simulink model "playback_data"  (R2015a)
settings: Solver=FixedStepDiscrete  SolverMode=SingleTasking  StartTime=76  StopTime=110  FixedStep=sample_time  RelTol=1e-3
undefined symbols (not defined in the file): A1_notch_f1, A2_notch_f1, A_kalman_swing_load, A_kalman_transverse, A_kalman_vertical, A_lpf_accelerometer, A_lpf_dtau, A_lpf_fourbar_angles, A_lpf_imu, A_lpf_lateral_angle, B1_lpf_accelerometer, B1_lpf_dtau, B1_lpf_fourbar_angles, B1_lpf_imu, B1_lpf_lateral_angle, B1_notch_f1, B2_lpf_accelerometer, B2_lpf_dtau, B2_lpf_fourbar_angles, B2_lpf_imu, B2_lpf_lateral_angle, B2_notch_f1, B_dx_versus_x0, B_kalman_swing_load, B_kalman_transverse, B_kalman_vertical, backwards_K_sag_of_t, backwards_P_sag_of_t, C_kalman_swing_load, C_kalman_transverse, C_kalman_vertical, com_leg_motor, com_torso, contact_threshold, control_start_time, d_ankle_to_foot, d_vertical_com, desired_com_forward_velocity, desired_com_lateral_velocity, desired_initial_leg_roll_left, desired_initial_leg_roll_right, desired_stance_beta2, desired_standing_torso_pitch, desired_standing_torso_roll, desired_standing_z, desired_torso_pitch, desired_torso_roll, Discrete, enable_bouncing, fcut_contact, fdesignblkfcn, forward_dx_of_dxstar, forward_x_of_dxstar, g, gcbh, HIP_MTR_MAX_CONT_TORQUE, HIP_MTR_MAX_TORQUE, i_leg_motor, i_robot, i_torso ... (+78)
libraries: simulink x65, dsparch4 x18, ctrlSharedLib x14, dspfdesign x4
(part 11 of 13)

== matlab function playback_data/Control1/Behavior Control/Primary and Lateral Behavior/Desired Forward Velocity ==
  data: dx_takeoff input; desired_dx output; desired_forward_velocity input; forward_velocity_target_step parameter
function desired_dx = dx_command(dx_takeoff, desired_forward_velocity, forward_velocity_target_step)
    desired_direction = sign(desired_forward_velocity);
    desired_dx = dx_takeoff + desired_direction*forward_velocity_target_step;
    desired_dx = max(min(desired_dx, abs(desired_forward_velocity)),-abs(desired_forward_velocity));
end

== matlab function playback_data/Control1/Behavior Control/Primary and Lateral Behavior/Flight/Avoid Hitting Mechanical Limits ==
  data: back_cmd output double; front_cmd output double; dback_cmd output double; dfront_cmd output double; ddback_cmd output double; ddfront_cmd output double; back_desired input; dback_desired input; ddback_desired input; front_desired input; dfront_desired input; ddfront_desired input; min_front_bar_angle parameter; max_front_bar_angle parameter; min_back_bar_angle parameter; max_back_bar_angle parameter
%% Avoid joint limits by ensuring we don't command velocities/accelerations that would push us into them when we are close to them.
function [back_cmd, front_cmd, dback_cmd, dfront_cmd, ddback_cmd, ddfront_cmd] ...
    = AvoidFourbarLimits(back_desired,dback_desired, ddback_desired, ...
          front_desired, dfront_desired, ddfront_desired, ...
          min_front_bar_angle, max_front_bar_angle, min_back_bar_angle, max_back_bar_angle)
    [back_cmd, front_cmd, dback_cmd, dfront_cmd, ddback_cmd, ddfront_cmd] = AvoidFourbarLimits(back_desired,dback_desired, ddback_desired, front_desired, dfront_desired, ddfront_desired, min_front_bar_angle, max_front_bar_angle, min_back_bar_angle, max_back_bar_angle);
end

== matlab function playback_data/Control1/Behavior Control/Primary and Lateral Behavior/Flight/Avoid Virtual Leg Length Limits ==
  data: l_leg_desired input; dl_leg_desired input; ddl_leg_desired input; l_leg_cmd output double; dl_leg_cmd output double; ddl_leg_cmd output double; min_leg_length parameter; max_leg_length parameter
%% Avoid virtual leg length limits by ensuring we don't command position/velocities/accelerations that would hit them.
function [l_leg_cmd, dl_leg_cmd, ddl_leg_cmd] = AvoidVirtualLengthLimits(l_leg_desired, dl_leg_desired, ddl_leg_desired, min_leg_length, max_leg_length)
    [l_leg_cmd, dl_leg_cmd, ddl_leg_cmd] = AvoidVirtualLengthLimits(l_leg_desired, dl_leg_desired, ddl_leg_desired, min_leg_length, max_leg_length);
end

== matlab function playback_data/Control1/Behavior Control/Primary and Lateral Behavior/Flight/Calculate Time Until Touchdown ==
  data: z_dz input; t output; z_land parameter; g parameter
function t = EstimateTouchdown(z_dz, z_land, g)
  z_hat = z_dz(1); 
  dz_hat = z_dz(2);
  t = (-dz_hat-sqrt( max(dz_hat^2 - 4*g/2*(z_land-z_hat),0) ))/(-g);
end

== matlab function playback_data/Control/Behavior Control/Primary and Lateral Behavior/Closed Loop Compensation/ESTIMATE CLOSED LOOP ERROR Y FOR VARIABLE SPEED ==
  data: dx_land_hist input; A_cl output; delta_ux_hist input; dx_lift_hist input; dx_star_hist input; B_dx_versus_x0 parameter; W_real input; epsilon_0 output; c output; A_cl_nb output; epsilon_0_nb output; c_nb output
function [A_cl, epsilon_0, c, ...
          A_cl_nb, epsilon_0_nb, c_nb] = error_fitting_dxstar...
         (dx_land_hist, delta_ux_hist, dx_lift_hist, dx_star_hist,...
          B_dx_versus_x0, W_real)
% data_length = min([length(dx_lift_hist), filter_length]);
data_length = length(dx_lift_hist);
assert(data_length < 100);
% add fake data
fake_dx_land_err_magnitude = 0.1; fake_dx_star_magnitude = 0.1;
[fgrid_dx_land_err, fgrid_dx_star, fgrid_dx_lift_err] = ...
    meshgrid(fake_dx_land_err_magnitude*[-1 1],fake_dx_star_magnitude*[-1 1],0);
fake_data_length = numel(fgrid_dx_land_err);
fake_dx_land_err = fgrid_dx_land_err(:);
fake_dx_star = fgrid_dx_star(:);
fake_dx_lift_err = fgrid_dx_lift_err(:);
fake_delta_ux = zeros(fake_data_length,1);
% assert(fake_data_length<100);
% assert(filter_length<100);
% fake_dx_land_err = linspace(-0.1, 0.1, fake_data_length)';
% fake_dx_lift_err = zeros(fake_data_length,1);
% fake_delta_ux = zeros(fake_data_length,1);
% fake_dx_star = linspace(-0.25, 0.25, fake_data_length)';
dx_land_err = [reshape(dx_land_hist(1:data_length)-dx_star_hist(1:data_length),...
                       data_length, 1); fake_dx_land_err];
dx_lift_err = [reshape(dx_lift_hist(1:data_length)-dx_star_hist(1:data_length),...
                       data_length, 1); fake_dx_lift_err];
dx_star = [reshape(dx_star_hist(1:data_length), data_length,1); fake_dx_star];
delta_ux = [reshape(delta_ux_hist(1:data_length), data_length, 1); fake_delta_ux];
% weighted least squares
W = diag([W_real*ones(1,data_length), ones(1,fake_data_length)]);
Y = dx_lift_err - B_dx_versus_x0*delta_ux;
X = [dx_land_err, dx_star, ones(data_length+fake_data_length,1)];
% linear regression for s_{i+1}-s0 = A_cl*(s_i-s0) + epsilon_0 + c(s0) + B*delta_u
% solve for Y = X*beta, beta column vector
beta_hat = (X'*W*X)\X'*W*Y;
W_nobias = diag([W_real*ones(1,data_length), 0.001*ones(1,fake_data_length)]);
beta_hat_nobias = (X'*W_nobias*X)\X'*W_nobias*Y;
A_cl = beta_hat(1);
c = beta_hat(2);
epsilon_0 = beta_hat(3);
A_cl_nb = beta_hat_nobias(1);
c_nb = beta_hat_nobias(2);
epsilon_0_nb = beta_hat_nobias(3);

== matlab function playback_data/Control/Behavior Control/Primary and Lateral Behavior/Desired Forward Velocity ==
  data: dx_takeoff input; desired_dx output; desired_forward_velocity input; forward_velocity_target_step parameter
function desired_dx = dx_command(dx_takeoff, desired_forward_velocity, forward_velocity_target_step)
    desired_direction = sign(desired_forward_velocity);
    desired_dx = dx_takeoff + desired_direction*forward_velocity_target_step;
    desired_dx = max(min(desired_dx, abs(desired_forward_velocity)),-abs(desired_forward_velocity));
end

== matlab function playback_data/Control/Behavior Control/Primary and Lateral Behavior/Flight/Avoid Hitting Mechanical Limits ==
  data: back_cmd output double; front_cmd output double; dback_cmd output double; dfront_cmd output double; ddback_cmd output double; ddfront_cmd output double; back_desired input; dback_desired input; ddback_desired input; front_desired input; dfront_desired input; ddfront_desired input; min_front_bar_angle parameter; max_front_bar_angle parameter; min_back_bar_angle parameter; max_back_bar_angle parameter
%% Avoid joint limits by ensuring we don't command velocities/accelerations that would push us into them when we are close to them.
function [back_cmd, front_cmd, dback_cmd, dfront_cmd, ddback_cmd, ddfront_cmd] ...
    = AvoidFourbarLimits(back_desired,dback_desired, ddback_desired, ...
          front_desired, dfront_desired, ddfront_desired, ...
          min_front_bar_angle, max_front_bar_angle, min_back_bar_angle, max_back_bar_angle)
    [back_cmd, front_cmd, dback_cmd, dfront_cmd, ddback_cmd, ddfront_cmd] = AvoidFourbarLimits(back_desired,dback_desired, ddback_desired, front_desired, dfront_desired, ddfront_desired, min_front_bar_angle, max_front_bar_angle, min_back_bar_angle, max_back_bar_angle);
end

== matlab function playback_data/Control/Behavior Control/Primary and Lateral Behavior/Flight/Avoid Virtual Leg Length Limits ==
  data: l_leg_desired input; dl_leg_desired input; ddl_leg_desired input; l_leg_cmd output double; dl_leg_cmd output double; ddl_leg_cmd output double; min_leg_length parameter; max_leg_length parameter
%% Avoid virtual leg length limits by ensuring we don't command position/velocities/accelerations that would hit them.
function [l_leg_cmd, dl_leg_cmd, ddl_leg_cmd] = AvoidVirtualLengthLimits(l_leg_desired, dl_leg_desired, ddl_leg_desired, min_leg_length, max_leg_length)
    [l_leg_cmd, dl_leg_cmd, ddl_leg_cmd] = AvoidVirtualLengthLimits(l_leg_desired, dl_leg_desired, ddl_leg_desired, min_leg_length, max_leg_length);
end

== matlab function playback_data/Control/Behavior Control/Primary and Lateral Behavior/Flight/Calculate Time Until Touchdown ==
  data: z_dz input; t output; z_land parameter; g parameter
function t = EstimateTouchdown(z_dz, z_land, g)
  z_hat = z_dz(1); 
  dz_hat = z_dz(2);
  t = (-dz_hat-sqrt( max(dz_hat^2 - 4*g/2*(z_land-z_hat),0) ))/(-g);
end

== matlab function playback_data/Control1/Behavior Control/Primary and Lateral Behavior/Flight/Convert COM Position to Joint Angles + Leg Length  ==
  data: hopping input; desired_leg_length output; X_star input; Y_star input; Z_star input; right_left input; com_pelvis_body input; desired_alpha output; desired_beta output; dcom_pelvis_body input; roll input; pitch input; sagittal_angle input; lateral_angle input; leg_length input; lateral_offset parameter; desired_initial_leg_roll_right parameter; desired_initial_leg_roll_left parameter; d_vertical_com parameter; desired_standing_z parameter
function [ desired_leg_length, desired_alpha, desired_beta ]  =  ...
          ConvertToJointAnglesAndLegLength(hopping, X_star, Y_star, Z_star, right_left,...
                           com_pelvis_body, dcom_pelvis_body, ...
                           roll, pitch, sagittal_angle, lateral_angle, leg_length,...
                           lateral_offset, desired_initial_leg_roll_right, desired_initial_leg_roll_left, d_vertical_com, desired_standing_z) 

    q = [roll(1), pitch(1), sagittal_angle(1), lateral_angle(1), leg_length(1)];
    dq = [roll(2), pitch(2), sagittal_angle(2), lateral_angle(2), leg_length(2)];
    [desired_alpha, desired_beta, desired_leg_length]  =  ConvertComPositionToLegAnglesAndLegLength(X_star, Y_star, Z_star, right_left, com_pelvis_body, dcom_pelvis_body, q, dq, lateral_offset);   
                       
    if ~hopping
        desired_leg_length = [desired_standing_z-d_vertical_com; 0; 0];
        desired_alpha = [pi - pitch(1); -pitch(2); 0];
        desired_beta = [desired_initial_leg_roll_left; 0; 0];
        if right_left
            desired_beta = [desired_initial_leg_roll_right; 0; 0];
        end
    end
    
end

== matlab function playback_data/Control1/Behavior Control/Primary and Lateral Behavior/Flight/Generate Parabolic Foot Trajectories ==
  data: time_remaining input; est_duration input; x_star input; y_star input; x0 input; dx0 input; y0 input; dy0 input; zdz0 input; max_retract input; flight input; z_land parameter; min_f_duration parameter; X_star output size=3; Y_star output size=3; Z_star output size=3
%% Parabolic trajectory generation for x, y, and z
% est_duration: estimated flight time
% time_remaining: time until estimated touchdown
% stance: 1 if in stance, 0 otherwise
% x_star: desired x for foot to COM
% y_star: desired y for foot to COM
% x0: x position at takeoff
% y0: y position at takeoff
% zdz0: [z, dz] at takeoff
% max_retract: how high to lift z for ground clearance
% z_land: nominal z height for landing
% min_f_duration: minimum trajectory time

function [X_star, Y_star, Z_star]  =  ...
          GenerateParabolicFootTrajectory(time_remaining, est_duration,  ...
                               x_star, y_star, x0, dx0, y0, dy0, zdz0, ...
                               max_retract,  flight, z_land, min_f_duration)

if ~flight
    X_star = [0;0;0];
    Y_star = [0;0;0];
    Z_star = [0;0;0];
    return;
end
                           
% we are solving for yawed coordinates xyz of com-foot in flight and
% converting them to joint angles

% estimate z ballistically
% z = z_dz_liftoff(1) + z_dz_liftoff(2)*t_flight -g/2*t_flight^2;
% dz = z_dz_liftoff(2) - g*t_flight;
% 
% z = com_xdx_ydy_zdz(5); dz = com_xdx_ydy_zdz(6);
% time_remaining = (-dz-sqrt(max(dz^2 - 4*g/2*(z_land-z), 0) ) )/ (-g); % ballistic estimate of landing


  % plan a traj from init to desired in estimated duration. Use a
  % discontinuous initial condition if estimated duration too short.
  duration = max(est_duration, min_f_duration);
  t_r = max(min(time_remaining, duration),0);
  % sweep a parabola from x0 to x_star with dx_end = -dx0
  dx_star = dx0;
  x_star_t = x_star + dx_star*t_r + (x0-x_star-dx_star*duration)*(t_r/duration)^2;
  dx_star_t = -dx_star - 2*(x0-x_star-dx_star*duration)*(t_r/duration^2);
  ddx_star_t =  2*(x0-x_star-dx_star*duration)*(1/duration^2);
  
  % same for y
  dy_star = dy0;
  y_star_t = y_star + dy_star*t_r + (y0-y_star-dy_star*duration)*(t_r/duration)^2;
  dy_star_t = -dy_star - 2*(y0-y_star-dy_star*duration)*(t_r/duration^2);
  ddy_star_t =  2*(y0-y_star-dy_star*duration)*(1/duration^2);
  
  % Zero out velocities when out of time
  if time_remaining < 0
    dx_star_t = 0; ddx_star_t = 0;
    dy_star_t = 0; ddy_star_t = 0;
  end 
  
  % split duration into thirds.  First segment: parabola from z0 to
  % max_retract.  Second and third segments, cos to landing.
  z0 = zdz0(1);
  dt3 = duration / 3;
  z_min = z_land - max_retract;
  if t_r > 2*dt3;
    z_star_t = z_min + (z0-z_min)*((t_r-2*dt3)/dt3)^2;
    dz_star_t = -(z0-z_min)*2*(t_r-2*dt3)/dt3/dt3;
    ddz_star_t = (z0-z_min)*2/dt3^2;
  else
    z_star_t = z_land + (z_min-z_land)/2*(1-cos(t_r/(2*dt3)*pi));
    dz_star_t = -(z_min-z_land)/2*sin(t_r/(2*dt3)*pi)*pi/(2*dt3);
    ddz_star_t = (z_min-z_land)/2*cos(t_r/(2*dt3)*pi)*(pi/(2*dt3))^2;
  end
  
  % track a sinusoidal z of amplitude max_retract, finishing a half-cycle by t_end
  X_star = [x_star_t; dx_star_t; ddx_star_t];
  Y_star = [y_star_t; dy_star_t; ddy_star_t];
  Z_star = [z_star_t; dz_star_t; ddz_star_t];

== matlab function playback_data/Control1/Behavior Control/Primary and Lateral Behavior/Flight/Lateral Flight Control ==
  data: hopping input; tau_primary output; tau_secondary output; RightLeftPrimary input; TorsoRoll input; LLegRoll input; RLegRoll input; Beta1_star input; Roll_star input; K_right_lat_flight parameter; K_left_lat_flight parameter; K_right_lat_flight_winch parameter; K_left_lat_flight_winch parameter; Q_phibeta1beta2 parameter; Q_phibeta1beta2_winch parameter; m_torso parameter; m_leg_motor parameter; com_torso parameter; i_torso parameter; i_leg_motor parameter; g parameter; lateral_offset parameter; adjusted_ref output; feedforward output; desired_initial_leg_roll_left parameter; desired_initial_leg_roll_right parameter
% full_state = [Roll; Beta1; Beta2; dRoll; dBeta1; dBeta2];
function [tau_primary, tau_secondary, ...
          adjusted_ref, feedforward] = lateral_flight_control(hopping, RightLeftPrimary,...
          TorsoRoll, LLegRoll, RLegRoll, Beta1_star, Roll_star,...
          K_right_lat_flight, K_left_lat_flight, K_right_lat_flight_winch, K_left_lat_flight_winch, Q_phibeta1beta2, Q_phibeta1beta2_winch,...
          m_torso, m_leg_motor, com_torso, i_torso, i_leg_motor, g, lateral_offset, desired_initial_leg_roll_left, desired_initial_leg_roll_right)

    d = norm(com_torso(2:3));
    It_f = i_torso(1);
    Im_f = i_leg_motor(1); 
    phidphi = TorsoRoll; 
    symdsym = LLegRoll-RLegRoll;
    ang_mom = phidphi(2)*(m_torso*d^2 + It_f + 2*(m_leg_motor*lateral_offset^2+ Im_f)) -symdsym(2)*(m_leg_motor*lateral_offset^2+Im_f);

    if RightLeftPrimary == 1
        Beta1 = RLegRoll;
        Beta2 = LLegRoll;
        Beta2_star = [desired_initial_leg_roll_left; 0; 0];
    else
        Beta1 = LLegRoll;
        Beta2 = RLegRoll;
        Beta2_star = [desired_initial_leg_roll_right; 0; 0];
    end    
    
    if ~hopping
        Q_phibeta1beta2 = Q_phibeta1beta2_winch;
        K_right_lat_flight = K_right_lat_flight_winch;
        K_left_lat_flight = K_left_lat_flight_winch;
    end

    ref_old = [Roll_star(1); Beta1_star(1); Beta2_star(1)];
    dref_old = [0; Beta1_star(2); Beta2_star(2)];
    ddref_old = [0; Beta1_star(3); Beta2_star(3)];
    
    % eliminate beta2 from state using momentum:
    % s_old = T*s_new+D(t); s_new = [phi; beta1];
    % dbeta_R = L/(Im_f+mm*r^2) - (It_f+mm*d^2+2*Im_f+2*mm*r^2)/(Im_f+mm*r^2)*dphi + dbeta_L 
    % beta_R = beta_R0 + L/(Im_f+mm*r^2)*t - ((It_f+mm*d^2+2*Im_f+2*mm*r^2)/(Im_f+mm*r^2)*(phi-phi0) + (beta_L-beta_L0)
    % beta_R = [beta_R0-b1*phi0-b2*beta_L0 + a*t + b1*phi + b2*beta_L;
    
    if RightLeftPrimary == 1 % beta_2 is beta_L, beta_1 is beta_R, eliminate beta2
      a = -ang_mom/(Im_f+m_leg_motor*lateral_offset^2);
      b1 = (It_f+m_torso*d^2+2*Im_f+2*m_leg_motor*lateral_offset^2)/(Im_f+m_leg_motor*lateral_offset^2); b2 = 1;
    else
      a = +ang_mom/(Im_f+m_leg_motor*lateral_offset^2);
      b1 = -(It_f+m_torso*d^2+2*Im_f+2*m_leg_motor*lateral_offset^2)/(Im_f+m_leg_motor*lateral_offset^2); b2 = 1;
    end
    
    T = [eye(2); b1, b2];
    %  D = [0; 0; 0; 0; beta_R0 - b1*phi0 - b2*beta_L0 + a*t; a];
    D = [0;0; Beta2(1) - b1*phidphi(1) - b2*Beta1(1)];
    
    % old cost (state s)  (s-s_ref)' * Q *(s-s_ref);
    % new cost (state r) =(T*r+D-s_ref)'*Q*(T*r+D-s_ref);
    %                    =(r+ (T'QT)^{-1}T'Q(D-s_ref))'*T'QT*
    %                     (r + (T'QT)^{-1}T'Q(D-s_ref))
    
    
    Q_new = T'*Q_phibeta1beta2*T;
    ref_new = Q_new\T'*Q_phibeta1beta2*(ref_old-D);
    ref_new_vel = Q_new\T'*Q_phibeta1beta2*(dref_old - [0;0; a]);
    ref_accels = Q_new\T'*Q_phibeta1beta2*(ddref_old);

    % A_phidphi_betadbeta1 = [0 1 0 0; 0 0 0 0; 0 0 0 1; 0 0 0 0];
    % assume beta1 is right
    if RightLeftPrimary == 1
        B_new_state = [0 0; 0 0; -1/(It_f+m_torso*d^2), 1/(It_f+m_torso*d^2); 1/(It_f+m_torso*d^2)+1/(Im_f+m_leg_motor*lateral_offset^2), -1/(It_f+m_torso*d^2)];
    else
        B_new_state = [0 0; 0 0; 1/(It_f+m_torso*d^2), -1/(It_f+m_torso*d^2); 1/(It_f+m_torso*d^2)+1/(Im_f+m_leg_motor*lateral_offset^2), -1/(It_f+m_torso*d^2)];
    end      
    
    %   K = lqr(A_phidphi_betadbeta1, B_phidphi_betadbeta1, Q_new, R_lat_flight);
    if RightLeftPrimary == 1
      K = K_right_lat_flight;
    else
      K = K_left_lat_flight;
    end

    new_state = [phidphi(1); Beta1(1); phidphi(2); Beta1(2)];
    new_ref_traj = [ref_new; ref_new_vel];

    feedforward = B_new_state([3 4],:)\ref_accels;
    if ~hopping, feedforward = -(m_leg_motor)*g*lateral_offset*ones(2,1); end
    tau_lqr = feedforward - K*(new_state-new_ref_traj);
    tau_1 = tau_lqr(1); tau_2 = tau_lqr(2);
    implied_beta2_star = [0 0 1]*(T*ref_new+D);
    implied_dbeta2_star = [0 0 1]*(T*ref_new_vel+[0; 0; a]);
    % implied_betadbeta2_star = [0 0 0 0 1 0; 0 0 0 0 0 1]*(T*ref_new+D);
    adjusted_ref = [ref_new; implied_beta2_star; ref_new_vel; implied_dbeta2_star];

    tau_primary = tau_1;
    tau_secondary = tau_2;

== matlab function playback_data/Control/Behavior Control/Primary and Lateral Behavior/Flight/Convert COM Position to Joint Angles + Leg Length  ==
  data: hopping input; desired_leg_length output; X_star input; Y_star input; Z_star input; right_left input; com_pelvis_body input; desired_alpha output; desired_beta output; dcom_pelvis_body input; roll input; pitch input; sagittal_angle input; lateral_angle input; leg_length input; lateral_offset parameter; desired_initial_leg_roll_right parameter; desired_initial_leg_roll_left parameter; d_vertical_com parameter; desired_standing_z parameter
function [ desired_leg_length, desired_alpha, desired_beta ]  =  ...
          ConvertToJointAnglesAndLegLength(hopping, X_star, Y_star, Z_star, right_left,...
                           com_pelvis_body, dcom_pelvis_body, ...
                           roll, pitch, sagittal_angle, lateral_angle, leg_length,...
                           lateral_offset, desired_initial_leg_roll_right, desired_initial_leg_roll_left, d_vertical_com, desired_standing_z) 

    q = [roll(1), pitch(1), sagittal_angle(1), lateral_angle(1), leg_length(1)];
    dq = [roll(2), pitch(2), sagittal_angle(2), lateral_angle(2), leg_length(2)];
    [desired_alpha, desired_beta, desired_leg_length]  =  ConvertComPositionToLegAnglesAndLegLength(X_star, Y_star, Z_star, right_left, com_pelvis_body, dcom_pelvis_body, q, dq, lateral_offset);   
                       
    if ~hopping
        desired_leg_length = [desired_standing_z-d_vertical_com; 0; 0];
        desired_alpha = [pi - pitch(1); -pitch(2); 0];
        desired_beta = [desired_initial_leg_roll_left; 0; 0];
        if right_left
            desired_beta = [desired_initial_leg_roll_right; 0; 0];
        end
    end
    
end

== matlab function playback_data/Control/Behavior Control/Primary and Lateral Behavior/Flight/Generate Parabolic Foot Trajectories ==
  data: time_remaining input; est_duration input; x_star input; y_star input; x0 input; dx0 input; y0 input; dy0 input; zdz0 input; max_retract input; flight input; z_land parameter; min_f_duration parameter; X_star output size=3; Y_star output size=3; Z_star output size=3
%% Parabolic trajectory generation for x, y, and z
% est_duration: estimated flight time
% time_remaining: time until estimated touchdown
% stance: 1 if in stance, 0 otherwise
% x_star: desired x for foot to COM
% y_star: desired y for foot to COM
% x0: x position at takeoff
% y0: y position at takeoff
% zdz0: [z, dz] at takeoff
% max_retract: how high to lift z for ground clearance
% z_land: nominal z height for landing
% min_f_duration: minimum trajectory time

function [X_star, Y_star, Z_star]  =  ...
          GenerateParabolicFootTrajectory(time_remaining, est_duration,  ...
                               x_star, y_star, x0, dx0, y0, dy0, zdz0, ...
                               max_retract,  flight, z_land, min_f_duration)

if ~flight
    X_star = [0;0;0];
    Y_star = [0;0;0];
    Z_star = [0;0;0];
    return;
end
                           
% we are solving for yawed coordinates xyz of com-foot in flight and
% converting them to joint angles

% estimate z ballistically
% z = z_dz_liftoff(1) + z_dz_liftoff(2)*t_flight -g/2*t_flight^2;
% dz = z_dz_liftoff(2) - g*t_flight;
% 
% z = com_xdx_ydy_zdz(5); dz = com_xdx_ydy_zdz(6);
% time_remaining = (-dz-sqrt(max(dz^2 - 4*g/2*(z_land-z), 0) ) )/ (-g); % ballistic estimate of landing


  % plan a traj from init to desired in estimated duration. Use a
  % discontinuous initial condition if estimated duration too short.
  duration = max(est_duration, min_f_duration);
  t_r = max(min(time_remaining, duration),0);
  % sweep a parabola from x0 to x_star with dx_end = -dx0
  dx_star = dx0;
  x_star_t = x_star + dx_star*t_r + (x0-x_star-dx_star*duration)*(t_r/duration)^2;
  dx_star_t = -dx_star - 2*(x0-x_star-dx_star*duration)*(t_r/duration^2);
  ddx_star_t =  2*(x0-x_star-dx_star*duration)*(1/duration^2);
  
  % same for y
  dy_star = dy0;
  y_star_t = y_star + dy_star*t_r + (y0-y_star-dy_star*duration)*(t_r/duration)^2;
  dy_star_t = -dy_star - 2*(y0-y_star-dy_star*duration)*(t_r/duration^2);
  ddy_star_t =  2*(y0-y_star-dy_star*duration)*(1/duration^2);
  
  % Zero out velocities when out of time
  if time_remaining < 0
    dx_star_t = 0; ddx_star_t = 0;
    dy_star_t = 0; ddy_star_t = 0;
  end 
  
  % split duration into thirds.  First segment: parabola from z0 to
  % max_retract.  Second and third segments, cos to landing.
  z0 = zdz0(1);
  dt3 = duration / 3;
  z_min = z_land - max_retract;
  if t_r > 2*dt3;
    z_star_t = z_min + (z0-z_min)*((t_r-2*dt3)/dt3)^2;
    dz_star_t = -(z0-z_min)*2*(t_r-2*dt3)/dt3/dt3;
    ddz_star_t = (z0-z_min)*2/dt3^2;
  else
    z_star_t = z_land + (z_min-z_land)/2*(1-cos(t_r/(2*dt3)*pi));
    dz_star_t = -(z_min-z_land)/2*sin(t_r/(2*dt3)*pi)*pi/(2*dt3);
    ddz_star_t = (z_min-z_land)/2*cos(t_r/(2*dt3)*pi)*(pi/(2*dt3))^2;
  end
  
  % track a sinusoidal z of amplitude max_retract, finishing a half-cycle by t_end
  X_star = [x_star_t; dx_star_t; ddx_star_t];
  Y_star = [y_star_t; dy_star_t; ddy_star_t];
  Z_star = [z_star_t; dz_star_t; ddz_star_t];

== matlab function playback_data/Control/Behavior Control/Primary and Lateral Behavior/Flight/Lateral Flight Control ==
  data: hopping input; tau_primary output; tau_secondary output; RightLeftPrimary input; TorsoRoll input; LLegRoll input; RLegRoll input; Beta1_star input; Roll_star input; K_right_lat_flight parameter; K_left_lat_flight parameter; K_right_lat_flight_winch parameter; K_left_lat_flight_winch parameter; Q_phibeta1beta2 parameter; Q_phibeta1beta2_winch parameter; m_torso parameter; m_leg_motor parameter; com_torso parameter; i_torso parameter; i_leg_motor parameter; g parameter; lateral_offset parameter; adjusted_ref output; feedforward output; desired_initial_leg_roll_left parameter; desired_initial_leg_roll_right parameter
% full_state = [Roll; Beta1; Beta2; dRoll; dBeta1; dBeta2];
function [tau_primary, tau_secondary, ...
          adjusted_ref, feedforward] = lateral_flight_control(hopping, RightLeftPrimary,...
          TorsoRoll, LLegRoll, RLegRoll, Beta1_star, Roll_star,...
          K_right_lat_flight, K_left_lat_flight, K_right_lat_flight_winch, K_left_lat_flight_winch, Q_phibeta1beta2, Q_phibeta1beta2_winch,...
          m_torso, m_leg_motor, com_torso, i_torso, i_leg_motor, g, lateral_offset, desired_initial_leg_roll_left, desired_initial_leg_roll_right)

    d = norm(com_torso(2:3));
    It_f = i_torso(1);
    Im_f = i_leg_motor(1); 
    phidphi = TorsoRoll; 
    symdsym = LLegRoll-RLegRoll;
    ang_mom = phidphi(2)*(m_torso*d^2 + It_f + 2*(m_leg_motor*lateral_offset^2+ Im_f)) -symdsym(2)*(m_leg_motor*lateral_offset^2+Im_f);

    if RightLeftPrimary == 1
        Beta1 = RLegRoll;
        Beta2 = LLegRoll;
        Beta2_star = [desired_initial_leg_roll_left; 0; 0];
    else
        Beta1 = LLegRoll;
        Beta2 = RLegRoll;
        Beta2_star = [desired_initial_leg_roll_right; 0; 0];
    end    
    
    if ~hopping
        Q_phibeta1beta2 = Q_phibeta1beta2_winch;
        K_right_lat_flight = K_right_lat_flight_winch;
        K_left_lat_flight = K_left_lat_flight_winch;
    end

    ref_old = [Roll_star(1); Beta1_star(1); Beta2_star(1)];
    dref_old = [0; Beta1_star(2); Beta2_star(2)];
    ddref_old = [0; Beta1_star(3); Beta2_star(3)];
    
    % eliminate beta2 from state using momentum:
    % s_old = T*s_new+D(t); s_new = [phi; beta1];
    % dbeta_R = L/(Im_f+mm*r^2) - (It_f+mm*d^2+2*Im_f+2*mm*r^2)/(Im_f+mm*r^2)*dphi + dbeta_L 
    % beta_R = beta_R0 + L/(Im_f+mm*r^2)*t - ((It_f+mm*d^2+2*Im_f+2*mm*r^2)/(Im_f+mm*r^2)*(phi-phi0) + (beta_L-beta_L0)
    % beta_R = [beta_R0-b1*phi0-b2*beta_L0 + a*t + b1*phi + b2*beta_L;
    
    if RightLeftPrimary == 1 % beta_2 is beta_L, beta_1 is beta_R, eliminate beta2
      a = -ang_mom/(Im_f+m_leg_motor*lateral_offset^2);
      b1 = (It_f+m_torso*d^2+2*Im_f+2*m_leg_motor*lateral_offset^2)/(Im_f+m_leg_motor*lateral_offset^2); b2 = 1;
    else
      a = +ang_mom/(Im_f+m_leg_motor*lateral_offset^2);
      b1 = -(It_f+m_torso*d^2+2*Im_f+2*m_leg_motor*lateral_offset^2)/(Im_f+m_leg_motor*lateral_offset^2); b2 = 1;
    end
    
    T = [eye(2); b1, b2];
    %  D = [0; 0; 0; 0; beta_R0 - b1*phi0 - b2*beta_L0 + a*t; a];
    D = [0;0; Beta2(1) - b1*phidphi(1) - b2*Beta1(1)];
    
    % old cost (state s)  (s-s_ref)' * Q *(s-s_ref);
    % new cost (state r) =(T*r+D-s_ref)'*Q*(T*r+D-s_ref);
    %                    =(r+ (T'QT)^{-1}T'Q(D-s_ref))'*T'QT*
    %                     (r + (T'QT)^{-1}T'Q(D-s_ref))
    
    
    Q_new = T'*Q_phibeta1beta2*T;
    ref_new = Q_new\T'*Q_phibeta1beta2*(ref_old-D);
    ref_new_vel = Q_new\T'*Q_phibeta1beta2*(dref_old - [0;0; a]);
    ref_accels = Q_new\T'*Q_phibeta1beta2*(ddref_old);

    % A_phidphi_betadbeta1 = [0 1 0 0; 0 0 0 0; 0 0 0 1; 0 0 0 0];
    % assume beta1 is right
    if RightLeftPrimary == 1
        B_new_state = [0 0; 0 0; -1/(It_f+m_torso*d^2), 1/(It_f+m_torso*d^2); 1/(It_f+m_torso*d^2)+1/(Im_f+m_leg_motor*lateral_offset^2), -1/(It_f+m_torso*d^2)];
    else
        B_new_state = [0 0; 0 0; 1/(It_f+m_torso*d^2), -1/(It_f+m_torso*d^2); 1/(It_f+m_torso*d^2)+1/(Im_f+m_leg_motor*lateral_offset^2), -1/(It_f+m_torso*d^2)];
    end      
    
    %   K = lqr(A_phidphi_betadbeta1, B_phidphi_betadbeta1, Q_new, R_lat_flight);
    if RightLeftPrimary == 1
      K = K_right_lat_flight;
    else
      K = K_left_lat_flight;
    end

    new_state = [phidphi(1); Beta1(1); phidphi(2); Beta1(2)];
    new_ref_traj = [ref_new; ref_new_vel];

    feedforward = B_new_state([3 4],:)\ref_accels;
    if ~hopping, feedforward = -(m_leg_motor)*g*lateral_offset*ones(2,1); end
    tau_lqr = feedforward - K*(new_state-new_ref_traj);
    tau_1 = tau_lqr(1); tau_2 = tau_lqr(2);
    implied_beta2_star = [0 0 1]*(T*ref_new+D);
    implied_dbeta2_star = [0 0 1]*(T*ref_new_vel+[0; 0; a]);
    % implied_betadbeta2_star = [0 0 0 0 1 0; 0 0 0 0 0 1]*(T*ref_new+D);
    adjusted_ref = [ref_new; implied_beta2_star; ref_new_vel; implied_dbeta2_star];

    tau_primary = tau_1;
    tau_secondary = tau_2;

== matlab function playback_data/Control/Behavior Control/Primary and Lateral Behavior/Flight/Virtual Leg to Four Bar ==
  data: l_leg input; dl_leg input; ddl_leg input; phi input; dphi input; ddphi input; back output; dback output; ddback output; front output; dfront output; ddfront output
function [back, dback, ddback, front, dfront, ddfront] = VirtualLegToFourBar(l_leg, dl_leg, ddl_leg, phi, dphi, ddphi)
    [back, dback, ddback, front, dfront, ddfront] = VirtualLegToFourBar(l_leg, dl_leg, ddl_leg, phi, dphi, ddphi);
end

== matlab function playback_data/Control/Behavior Control/Primary and Lateral Behavior/Stance/3D Inverse Dynamics yawed ==
  data: right_or_left input; primary_leg_torque output double size=1; primary_leg_force output double size=1; torso_roll input double size=2; torso_pitch input double size=2; torso_yaw input size=2; primary_sagittal_leg_angle input size=2; primary_leg_length input size=2; primary_leg_roll input size=2; secondary_leg_roll input size=2; GRF_desired input double size=3; ddRoll_desired input double size=1; g parameter; primary_lateral_torque output double size=1; secondary_lateral_torque output double size=1; m_leg_motor parameter; m_torso parameter; i_torso parameter; i_leg_motor parameter; lateral_offset parameter; com_torso parameter; torso_centerline_roll_offset_angle parameter
%% Inverse dynamics
function [primary_leg_torque, primary_leg_force, primary_lateral_torque, secondary_lateral_torque]  =  InverseDynamics3D(right_or_left,...
                                                                                                                         torso_roll, torso_pitch, torso_yaw, ...
                                                                                                                         primary_sagittal_leg_angle, primary_leg_length, ...
                                                                                                                         primary_leg_roll, secondary_leg_roll, ...
                                                                                                                         GRF_desired, ddRoll_desired, ...
                                                                                                                         g, m_leg_motor, m_torso, i_torso, i_leg_motor, lateral_offset, com_torso, torso_centerline_roll_offset_angle)

    d = norm(com_torso(2:3));
    It = mean(i_torso);
    Im = mean(i_leg_motor);
    
    phi    = torso_roll(1) + torso_centerline_roll_offset_angle; % roll
    theta  = torso_pitch(1);                   % pitch
    alpha1 = primary_sagittal_leg_angle(1);    % primary sagittal leg angle
    beta1  = primary_leg_roll(1);              % primary leg roll
    beta2  = secondary_leg_roll(1);            % secondary leg roll
    if right_or_left
        beta1 = beta1 - torso_centerline_roll_offset_angle;
        beta2 = beta2 + torso_centerline_roll_offset_angle;
    else
        beta1 = beta1 + torso_centerline_roll_offset_angle;
        beta2 = beta2 - torso_centerline_roll_offset_angle;
    end 
    l1     = primary_leg_length(1);            % primary leg length
    
    dphi    = torso_roll(2);
    dtheta  = torso_pitch(2);
    dpsi    = torso_yaw(2);
    dalpha1 = primary_sagittal_leg_angle(2);
    dbeta1  = primary_leg_roll(2);
    dbeta2  = secondary_leg_roll(2);
    dl1     = primary_leg_length(2);

    Fx = GRF_desired(1);
    Fy = GRF_desired(2);
    Fz = GRF_desired(3);
    ddphi = ddRoll_desired;

    if right_or_left == 1
      A = A_id_roll_yawed_right(lateral_offset,d,m_leg_motor,m_torso,It,Im,phi,theta,alpha1,beta1,beta2,l1);     
      B = B_id_roll_yawed_right(lateral_offset,d,g,m_leg_motor,m_torso,It,Im,phi,theta,alpha1,beta1,beta2,l1,dphi,dtheta,dpsi,dalpha1,dbeta1,dbeta2,dl1,Fx,Fy,Fz,ddphi);
    else
      A = A_id_roll_yawed_left(lateral_offset,d,m_leg_motor,m_torso,It,Im,phi,theta,alpha1,beta1,beta2,l1);     
      B = B_id_roll_yawed_left(lateral_offset,d,g,m_leg_motor,m_torso,It,Im,phi,theta,alpha1,beta1,beta2,l1,dphi,dtheta,dpsi,dalpha1,dbeta1,dbeta2,dl1,Fx,Fy,Fz,ddphi);
    end        
    
    x_id_roll = A \ B;
    primary_leg_torque = x_id_roll(10);
    primary_lateral_torque = x_id_roll(11);
    secondary_lateral_torque = x_id_roll(12);
    primary_leg_force = x_id_roll(13);
end

== matlab function playback_data/Control/Behavior Control/Primary and Lateral Behavior/Stance/COM X,Y,Z  trajectory generation ==
  data: stance input; hopping input; bouncing input; x_0 output size=1; y_0 output size=1; z_ref output size=1; dz_ref output size=1; ddz_ref output size=1; x_ref output size=1; dx_ref output size=1; y_ref output size=1; dy_ref output size=1; t input size=1; dx0 input; dy0 input; target_DX input; target_DY input; z_rest_new parameter; z_amplitude parameter; spring_frequency parameter; phase_0 parameter; forward_x_of_dxstar parameter; forward_dx_of_dxstar parameter; target_dx_range parameter; T_s parameter; desired_standing_z parameter; standing_bounce_amplitude parameter; standing_bounce_w input; standing_bounce_dw input
%% COM trajectory generation for stance & foot placement for flight

% Outputs:
% x_0: desired x position for COM at touchdown
% y_0: desired y position for COM at touchdown
% [z_ref, dz_ref, ddz_ref]: reference trajectory for vertical
% [x_ref, dx_ref]: reference trajectory for forward
% [y_ref, dy_ref]: reference trajectory for lateral

% Inputs:
% t: time since touchdown
% dx0: touchdown x velocity
% dy0: touchdown y velocity
% target_DX: desired x velocity at takeoff
% s_duration: nominal stance time
% z_rest_new: z height of oscillation
% target_dx_range: full range of possible x velocities in lookup table
% forward_x_of_dxstar: master lookup table for x trajectories
% T_s: tabled vector from 0 to s_duration

function [x_0, y_0,...
          z_ref, dz_ref, ddz_ref, ...
          x_ref, dx_ref, y_ref, dy_ref] ...
          = ReferenceTrajectory(stance, hopping, bouncing, t, dx0, dy0, target_DX, target_DY, z_rest_new, z_amplitude, ...
            spring_frequency, phase_0, forward_x_of_dxstar, forward_dx_of_dxstar, ...
            target_dx_range, T_s,...
            desired_standing_z, standing_bounce_amplitude, standing_bounce_w, standing_bounce_dw)
    
    % Z trajectory 
    z_ref =  z_rest_new + z_amplitude*sin(spring_frequency*t+phase_0);
    dz_ref = z_amplitude*spring_frequency*cos(spring_frequency*t+phase_0);
    ddz_ref = -z_amplitude*spring_frequency^2*sin(spring_frequency*t+phase_0);
    
    % saturate t and initial velocity to reference library
    t_sat = max( min(t, T_s(end)), 0);

    % [X, dX] trajectory from 0 to s_duration
    forward_x_given_dxstar = squeeze(interp1(target_dx_range, forward_x_of_dxstar, target_DX));
    forward_dx_given_dxstar = squeeze(interp1(target_dx_range, forward_dx_of_dxstar, target_DX));

    dx0 = max( min(dx0, max(forward_dx_given_dxstar(:,1))), min(forward_dx_given_dxstar(:,1)) );
    x_ref  = interp2(T_s, forward_dx_given_dxstar(:,1), forward_x_given_dxstar, t_sat, dx0);
    dx_ref = interp2(T_s, forward_dx_given_dxstar(:,1), forward_dx_given_dxstar, t_sat, dx0);
    x_0 = interp1(forward_dx_given_dxstar(:,1), forward_x_given_dxstar(:,1), dx0);

    % [Y, dY] trajectory from 0 to s_duration
    % Y uses same library as X
    forward_y_given_dxstar = squeeze(interp1(target_dx_range, forward_x_of_dxstar, target_DY));
    forward_dy_given_dxstar = squeeze(interp1(target_dx_range, forward_dx_of_dxstar, target_DY));

    dy0 = max( min(dy0, max(forward_dy_given_dxstar(:,1))), min(forward_dy_given_dxstar(:,1)) );
    y_ref  = interp2(T_s, forward_dy_given_dxstar(:,1), forward_y_given_dxstar, t_sat, dy0);
    dy_ref = interp2(T_s, forward_dy_given_dxstar(:,1), forward_dy_given_dxstar, t_sat, dy0);
    y_0 = interp1(forward_dy_given_dxstar(:,1), forward_y_given_dxstar(:,1), dy0);
    
    if ~hopping && ~bouncing % Standing still
        z_ref = desired_standing_z;
        dz_ref = 0;
        ddz_ref = 0;
        x_ref = 0;
        dx_ref = 0;
        y_ref = 0;
        dy_ref =0;
    elseif ~hopping && bouncing % Bouncing while standing
        z_ref = z_rest_new + standing_bounce_amplitude*sin(t*standing_bounce_w);
        dz_ref = standing_bounce_amplitude*cos(t*standing_bounce_w)*(t*standing_bounce_dw + standing_bounce_w);
        ddz_ref = standing_bounce_amplitude*(2*standing_bounce_dw*cos(t*standing_bounce_w) - (t*standing_bounce_dw + standing_bounce_w)^2*sin(t*standing_bounce_w));
        x_ref = 0;
        dx_ref = 0;
        y_ref = 0;
        dy_ref =0;
    end
    if ~stance % Flight
        z_ref = 0;
        dz_ref = 0;
        ddz_ref = 0;
        x_ref = 0;
        dx_ref = 0;
        y_ref = 0;
        dy_ref =0;    
    end
  
end

== matlab function playback_data/Control1/Behavior Control/Primary and Lateral Behavior/Flight/Virtual Leg to Four Bar ==
  data: l_leg input; dl_leg input; ddl_leg input; phi input; dphi input; ddphi input; back output; dback output; ddback output; front output; dfront output; ddfront output
function [back, dback, ddback, front, dfront, ddfront] = VirtualLegToFourBar(l_leg, dl_leg, ddl_leg, phi, dphi, ddphi)
    [back, dback, ddback, front, dfront, ddfront] = VirtualLegToFourBar(l_leg, dl_leg, ddl_leg, phi, dphi, ddphi);
end

== matlab function playback_data/Control/Behavior Control/Primary and Lateral Behavior/Stance/Feedback for Lateral Stabilization ==
  data: Fy_desired output; neutral_feedforward_Fy output; hopping input; stance input; right_left input; rolldroll input; symdsym input; y_dy input; beta2dbeta2 input; z_dz input; GRF_measured input; secondary_lateral_torque_desired output double size=1; m_torso parameter; m_leg_motor parameter; m_leg parameter; lateral_offset parameter; com_torso parameter; i_torso parameter; i_leg_motor parameter; desired_standing_torso_roll parameter; desired_torso_roll parameter; desired_stance_beta2 parameter; angular_momentum output; k_stance_secondary_roll parameter; k_lateral_accel_for_torso_roll parameter; g parameter; m_total_real parameter
%  x_front = [y, roll, sym, dy, droll, L]; 
function [Fy_desired,neutral_feedforward_Fy, secondary_lateral_torque_desired, angular_momentum]  =  ...
    FrontalStabilization(hopping, stance, right_left, rolldroll, symdsym, y_dy, beta2dbeta2, z_dz, GRF_measured,...
           m_torso, m_leg_motor, m_leg, lateral_offset, com_torso, i_torso, i_leg_motor, ...
           desired_standing_torso_roll, desired_torso_roll, desired_stance_beta2, k_stance_secondary_roll, k_lateral_accel_for_torso_roll, g, m_total_real)
    
    % Angular momentum about the pelvis in the frontal plane
    d = norm(com_torso(2:3));
    It_f = i_torso(1);
    Im_f = i_leg_motor(1);
    lateral_robot_inertia = m_torso*d^2 + It_f + 2*(m_leg_motor*lateral_offset^2+ Im_f);
    angular_momentum = rolldroll(2)*lateral_robot_inertia - symdsym(2)*(m_leg_motor*lateral_offset^2+Im_f);
    
    % Feedforward GRFy for inverse dynamics
    neutral_feedforward_Fy = GRF_measured(3)*y_dy(1)/z_dz(1);
    
    % Desired states
    if hopping
        desired_torso_roll_state = [desired_torso_roll; 0]; 
    else
        desired_torso_roll_state = [desired_standing_torso_roll; 0];
    end
    desired_beta2_state = [desired_stance_beta2; 0];
    
    % Motor torque commands
    %ddz = GRF_measured(3) / m_total_real - g;
    %gravity_comp = (m_leg_motor+m_leg)*lateral_offset*ddz;
    secondary_lateral_torque_desired = k_stance_secondary_roll*(desired_beta2_state - beta2dbeta2);
    feedback_Fy = (lateral_robot_inertia * k_lateral_accel_for_torso_roll*(desired_torso_roll_state - rolldroll)) / z_dz(1);
    Fy_desired =  neutral_feedforward_Fy + feedback_Fy;
    Fy_desired = min(max(Fy_desired, -0.5*abs(GRF_measured(3))), 0.5*abs(GRF_measured(3)));
    
    if ~stance
        Fy_desired = 0;
        secondary_lateral_torque_desired = 0;
        neutral_feedforward_Fy = 0;
    end
end

== matlab function playback_data/Control/Behavior Control/Primary and Lateral Behavior/Stance/LQR Feedback for Desired Forward GRF ==
  data: hopping input; stance input; GRFx_desired output; netural_pitch_ff output; true_ff output; GRFx_lqr output; ddtheta_star output; ddtheta_star_neutral output; xdx input; thetadtheta input; zdz input; Fz_desired input; xdx_ref input size=2; theta_star input; K_sag input; P_sag input; measured_GRF input; Fx_disturbance input; i_robot parameter; cost_to_go output double size=1; ang_mom output; desired_standing_torso_pitch parameter; k_LQR_sagittal_infinite parameter; P_LQR_sagittal_infinite parameter
%% LQR for x state

% stance: 1 if in stance, 0 otherwise
% xdx: [ x from stance leg to COM, dx of COM]
% thetadtheta: [pitch, dpitch]
% zdz: [z of COM, dz of COM]
% Fz: Desired z GRF
% xdx_ref: [x, dx] current reference point for COM
% theta_star: desired torso pitch
% K_sag: time dependent LQR gain


% sagittal_state: [x, pitch, dx, dptich]
% theta_star: desired torso pitch


function [GRFx_desired, netural_pitch_ff, true_ff, GRFx_lqr, ddtheta_star, ddtheta_star_neutral, cost_to_go, ang_mom]  =  ...
    LQR_Sagittal(hopping, stance, xdx, thetadtheta, zdz, Fz_desired, xdx_ref, theta_star, K_sag, P_sag, measured_GRF, Fx_disturbance, i_robot,...
    desired_standing_torso_pitch, k_LQR_sagittal_infinite, P_LQR_sagittal_infinite)


    sagittal_state = [xdx(1); thetadtheta(1); xdx(2); thetadtheta(2)];
    netural_pitch_ff = measured_GRF(3)*xdx(1)/zdz(1);
    true_ff = measured_GRF(3)*xdx_ref(1)/zdz(1);
    
%     if hopping
%         sagittal_reference = [xdx_ref(1), theta_star, xdx_ref(2), 0]';
%         sagittal_error = (sagittal_state - sagittal_reference);
%         cost_to_go = 0.5*sagittal_error'*P_sag*sagittal_error;
%         GRFx_lqr = - K_sag*sagittal_error;
%         GRFx_desired = true_ff + GRFx_lqr;
%     else
        sagittal_reference = [xdx_ref(1), desired_standing_torso_pitch, xdx_ref(2), 0]';
        sagittal_error = (sagittal_state - sagittal_reference);
        cost_to_go = 0.5*sagittal_error'*P_LQR_sagittal_infinite*sagittal_error;
        %GRFx_desired = i_robot/zdz(1)*(150*(thetadtheta(1)-desired_standing_torso_pitch) + 30*thetadtheta(2)) + netural_pitch_ff;
        GRFx_lqr = - k_LQR_sagittal_infinite*sagittal_error;
        GRFx_desired = GRFx_lqr + true_ff;
%     end
    
    GRFx_desired = GRFx_desired - Fx_disturbance;
    GRFx_desired = min(max(GRFx_desired, -0.5*abs(measured_GRF(3))), 0.5*abs(measured_GRF(3))); % saturate to friction cone
    
    if stance == 0
      GRFx_lqr = 0;
      cost_to_go = 0;
      netural_pitch_ff = 0;
      true_ff = 0;
    end
    
    % quantities for logging
    ddtheta_star_neutral = -(GRFx_lqr)*zdz(1)/i_robot;
    ddtheta_star = -(GRFx_desired - netural_pitch_ff)*zdz(1)/i_robot;
    ang_mom = i_robot*thetadtheta(2);
end

== matlab function playback_data/Control1/Behavior Control/Primary and Lateral Behavior/Stance/3D Inverse Dynamics yawed ==
  data: right_or_left input; primary_leg_torque output double size=1; primary_leg_force output double size=1; torso_roll input double size=2; torso_pitch input double size=2; torso_yaw input size=2; primary_sagittal_leg_angle input size=2; primary_leg_length input size=2; primary_leg_roll input size=2; secondary_leg_roll input size=2; GRF_desired input double size=3; ddRoll_desired input double size=1; g parameter; primary_lateral_torque output double size=1; secondary_lateral_torque output double size=1; m_leg_motor parameter; m_torso parameter; i_torso parameter; i_leg_motor parameter; lateral_offset parameter; com_torso parameter; torso_centerline_roll_offset_angle parameter
%% Inverse dynamics
function [primary_leg_torque, primary_leg_force, primary_lateral_torque, secondary_lateral_torque]  =  InverseDynamics3D(right_or_left,...
                                                                                                                         torso_roll, torso_pitch, torso_yaw, ...
                                                                                                                         primary_sagittal_leg_angle, primary_leg_length, ...
                                                                                                                         primary_leg_roll, secondary_leg_roll, ...
                                                                                                                         GRF_desired, ddRoll_desired, ...
                                                                                                                         g, m_leg_motor, m_torso, i_torso, i_leg_motor, lateral_offset, com_torso, torso_centerline_roll_offset_angle)

    d = norm(com_torso(2:3));
    It = mean(i_torso);
    Im = mean(i_leg_motor);
    
    phi    = torso_roll(1) + torso_centerline_roll_offset_angle; % roll
    theta  = torso_pitch(1);                   % pitch
    alpha1 = primary_sagittal_leg_angle(1);    % primary sagittal leg angle
    beta1  = primary_leg_roll(1);              % primary leg roll
    beta2  = secondary_leg_roll(1);            % secondary leg roll
    if right_or_left
        beta1 = beta1 - torso_centerline_roll_offset_angle;
        beta2 = beta2 + torso_centerline_roll_offset_angle;
    else
        beta1 = beta1 + torso_centerline_roll_offset_angle;
        beta2 = beta2 - torso_centerline_roll_offset_angle;
    end 
    l1     = primary_leg_length(1);            % primary leg length
    
    dphi    = torso_roll(2);
    dtheta  = torso_pitch(2);
    dpsi    = torso_yaw(2);
    dalpha1 = primary_sagittal_leg_angle(2);
    dbeta1  = primary_leg_roll(2);
    dbeta2  = secondary_leg_roll(2);
    dl1     = primary_leg_length(2);

    Fx = GRF_desired(1);
    Fy = GRF_desired(2);
    Fz = GRF_desired(3);
    ddphi = ddRoll_desired;

    if right_or_left == 1
      A = A_id_roll_yawed_right(lateral_offset,d,m_leg_motor,m_torso,It,Im,phi,theta,alpha1,beta1,beta2,l1);     
      B = B_id_roll_yawed_right(lateral_offset,d,g,m_leg_motor,m_torso,It,Im,phi,theta,alpha1,beta1,beta2,l1,dphi,dtheta,dpsi,dalpha1,dbeta1,dbeta2,dl1,Fx,Fy,Fz,ddphi);
    else
      A = A_id_roll_yawed_left(lateral_offset,d,m_leg_motor,m_torso,It,Im,phi,theta,alpha1,beta1,beta2,l1);     
      B = B_id_roll_yawed_left(lateral_offset,d,g,m_leg_motor,m_torso,It,Im,phi,theta,alpha1,beta1,beta2,l1,dphi,dtheta,dpsi,dalpha1,dbeta1,dbeta2,dl1,Fx,Fy,Fz,ddphi);
    end        
    
    x_id_roll = A \ B;
    primary_leg_torque = x_id_roll(10);
    primary_lateral_torque = x_id_roll(11);
    secondary_lateral_torque = x_id_roll(12);
    primary_leg_force = x_id_roll(13);
end
